simulink model "ClarkAndParkTransforms_harness"  (R2020a)
settings: Solver=VariableStepAuto  StartTime=0.0  StopTime=0.05  RelTol=1e-3
model workspace (MAT data in the model file):
  Vmax = 1
  tol = 1e-09
libraries: ElectricalModelLib x4, simulink x4
settings Model: OrderedModelArguments=off  Creator=cleme  LastModifiedBy=cleme

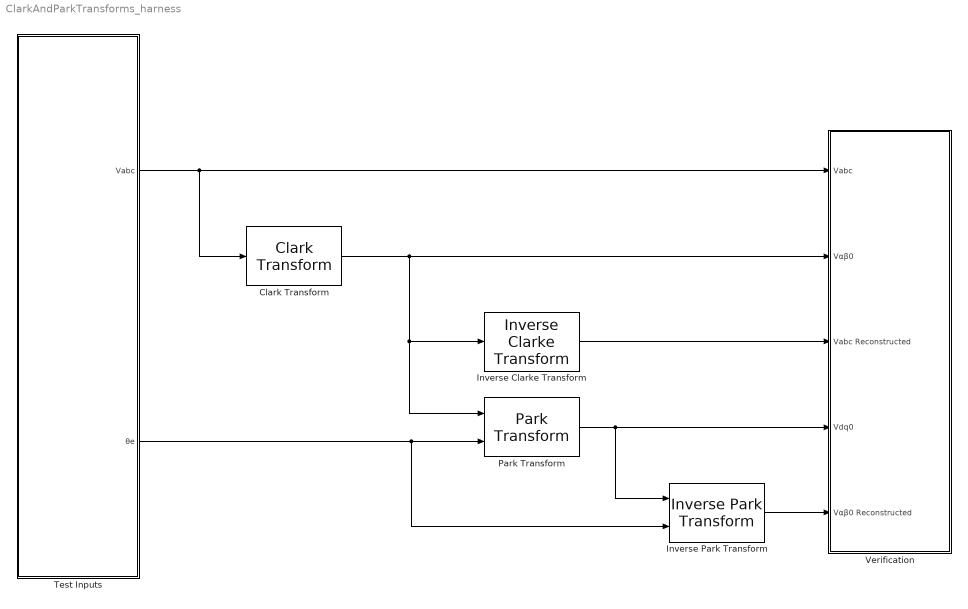
== system ClarkAndParkTransforms_harness ==
  Clark Transform : ElectricalModelLib/Clark Transform
  Inverse Clarke Transform : ElectricalModelLib/Inverse Clarke Transform
  Inverse Park Transform : ElectricalModelLib/Inverse Park Transform
  Park Transform : ElectricalModelLib/Park Transform
  Test Inputs : Subsystem
  Verification : Subsystem
  wires:
  Clark Transform/1 -> Park Transform/1, Inverse Clarke Transform/1, Verification/2(Vαβ0)
  Inverse Clarke Transform/1 -> Verification/3(Vabc Reconstructed)
  Test Inputs/1(Vabc) -> Clark Transform/1, Verification/1(Vabc)
  Test Inputs/2(θe) -> Inverse Park Transform/2, Park Transform/2
  Park Transform/1 -> Verification/4(Vdq0), Inverse Park Transform/1
  Inverse Park Transform/1 -> Verification/5(Vαβ0 Reconstructed)

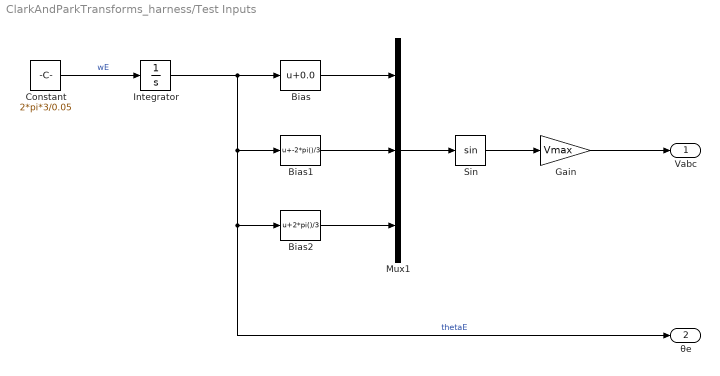
== system ClarkAndParkTransforms_harness/Test Inputs ==
  Bias : Bias  Bias=0.0
  Bias1 : Bias  Bias=-2*pi()/3
  Bias2 : Bias  Bias=2*pi()/3
  Constant : Constant  Value=2*pi*3/0.05
  Gain : Gain  Gain=Vmax
  Integrator : Integrator
  Mux1 : Mux  Inputs=3
  Sin : Trigonometry
  Vabc : Outport
  θe : Outport  Port=2
  wires:
  Sin/1 -> Gain/1
  Constant/1 -> Integrator/1  "wE"
  Integrator/1 -> θe/1, Bias2/1, Bias1/1, Bias/1  "thetaE"
  Bias2/1 -> Mux1/3
  Bias/1 -> Mux1/1
  Bias1/1 -> Mux1/2
  Mux1/1 -> Sin/1
  Gain/1 -> Vabc/1

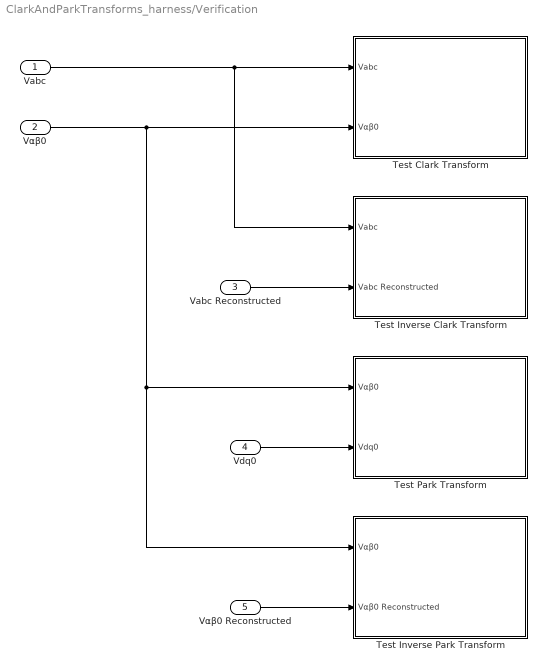
== system ClarkAndParkTransforms_harness/Verification ==
  Vabc : Inport
  Vαβ0 : Inport  Port=2
  Vabc Reconstructed : Inport  Port=3
  Vdq0 : Inport  Port=4
  Vαβ0 Reconstructed : Inport  Port=5
  Test Clark Transform : Subsystem
  Test Inverse Clark Transform : Subsystem
  Test Inverse Park Transform : Subsystem
  Test Park Transform : Subsystem
  wires:
  Vαβ0/1 -> Test Inverse Park Transform/1(Vαβ0), Test Park Transform/1(Vαβ0), Test Clark Transform/2(Vαβ0)
  Vabc/1 -> Test Clark Transform/1(Vabc), Test Inverse Clark Transform/1(Vabc)
  Vabc Reconstructed/1 -> Test Inverse Clark Transform/2(Vabc Reconstructed)
  Vαβ0 Reconstructed/1 -> Test Inverse Park Transform/2(Vαβ0 Reconstructed)
  Vdq0/1 -> Test Park Transform/2(Vdq0)

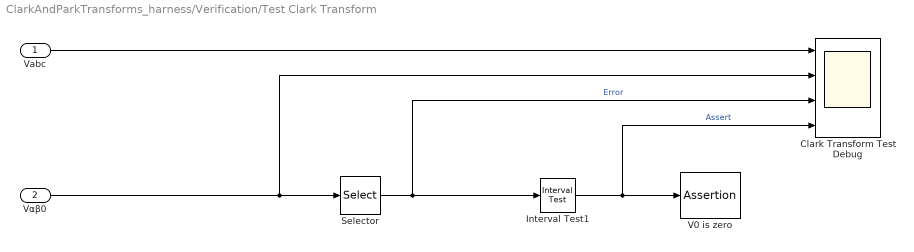
== system ClarkAndParkTransforms_harness/Verification/Test Clark Transform ==
  Vabc : Inport
  Vαβ0 : Inport  Port=2
  Clark Transform Test Debug : Scope  NumInputPorts=4
  Interval Test1 : simulink/Logic and Bit Operations/Interval Test  IntervalClosedRight=on  uplimit=tol  IntervalClosedLeft=on  lowlimit=-tol  OutDataTypeStr=boolean
      settings: AttributesFormatString=|
      | LB = %<lowlimit>
      | UB = %<uplimit>
  Selector : Selector  InputPortWidth=3  IndexOptions=Index vector (dialog)  Indices=3  OutputSizes=1
  V0 is zero : Assertion
  wires:
  Vabc/1 -> Clark Transform Test Debug/1
  Interval Test1/1 -> Clark Transform Test Debug/4, V0 is zero/1  "Assert"
  Vαβ0/1 -> Clark Transform Test Debug/2, Selector/1
  Selector/1 -> Interval Test1/1, Clark Transform Test Debug/3  "Error"

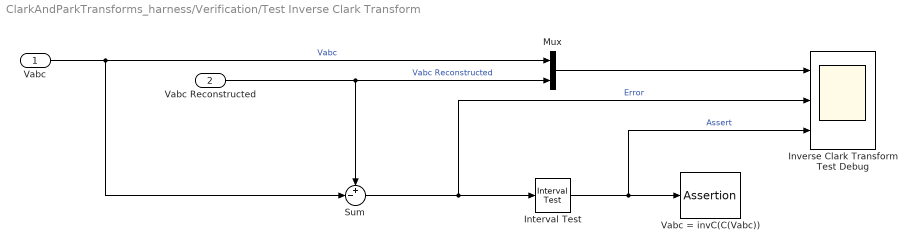
== system ClarkAndParkTransforms_harness/Verification/Test Inverse Clark Transform ==
  Vabc : Inport
  Vabc Reconstructed : Inport  Port=2
  Interval Test : simulink/Logic and Bit Operations/Interval Test  IntervalClosedRight=on  uplimit=tol  IntervalClosedLeft=on  lowlimit=-tol  OutDataTypeStr=boolean
      settings: AttributesFormatString=|
      | LB = %<lowlimit>
      | UB = %<uplimit>
  Inverse Clark Transform Test Debug : Scope  NumInputPorts=3
  Mux : Mux  Inputs=2
  Sum : Sum  Inputs=+-|
  "Vabc = invC(C(Vabc))  " : Assertion
  wires:
  Interval Test/1 -> Inverse Clark Transform Test Debug/3, "Vabc = invC(C(Vabc))  "/1  "Assert"
  Sum/1 -> Interval Test/1, Inverse Clark Transform Test Debug/2  "Error"
  Mux/1 -> Inverse Clark Transform Test Debug/1
  Vabc/1 -> Sum/2, Mux/1  "Vabc"
  Vabc Reconstructed/1 -> Sum/1, Mux/2  "Vabc Reconstructed"

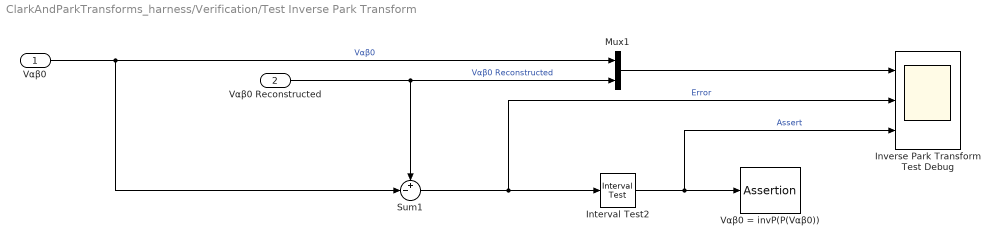
== system ClarkAndParkTransforms_harness/Verification/Test Inverse Park Transform ==
  Vαβ0 : Inport
  Vαβ0 Reconstructed : Inport  Port=2
  Interval Test2 : simulink/Logic and Bit Operations/Interval Test  IntervalClosedRight=on  uplimit=tol  IntervalClosedLeft=on  lowlimit=-tol  OutDataTypeStr=boolean
      settings: AttributesFormatString=|
      | LB = %<lowlimit>
      | UB = %<uplimit>
  Inverse Park Transform Test Debug : Scope  NumInputPorts=3
  Mux1 : Mux  Inputs=2
  Sum1 : Sum  Inputs=+-|
  Vαβ0 = invP(P(Vαβ0)) : Assertion
  wires:
  Interval Test2/1 -> Inverse Park Transform Test Debug/3, Vαβ0 = invP(P(Vαβ0))/1  "Assert"
  Vαβ0 Reconstructed/1 -> Sum1/1, Mux1/2  "Vαβ0 Reconstructed"
  Mux1/1 -> Inverse Park Transform Test Debug/1
  Vαβ0/1 -> Sum1/2, Mux1/1  "Vαβ0"
  Sum1/1 -> Inverse Park Transform Test Debug/2, Interval Test2/1  "Error"

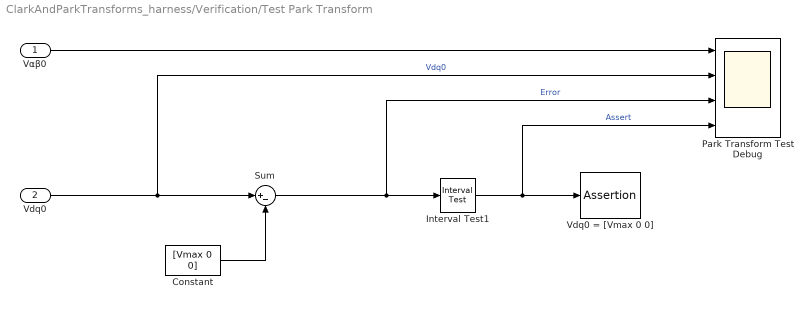
== system ClarkAndParkTransforms_harness/Verification/Test Park Transform ==
  Vαβ0 : Inport
  Vdq0 : Inport  Port=2
  Constant : Constant  Value=[Vmax 0 0]
  Interval Test1 : simulink/Logic and Bit Operations/Interval Test  IntervalClosedRight=on  uplimit=tol  IntervalClosedLeft=on  lowlimit=-tol  OutDataTypeStr=boolean
      settings: AttributesFormatString=|
      | LB = %<lowlimit>
      | UB = %<uplimit>
  Park Transform Test Debug : Scope  NumInputPorts=4
  Sum : Sum  Inputs=|+-
  Vdq0 = [Vmax 0 0] : Assertion
  wires:
  Vdq0/1 -> Sum/1, Park Transform Test Debug/2  "Vdq0"
  Interval Test1/1 -> Park Transform Test Debug/4, Vdq0 = [Vmax 0 0]/1  "Assert"
  Vαβ0/1 -> Park Transform Test Debug/1
  Sum/1 -> Park Transform Test Debug/3, Interval Test1/1  "Error"
  Constant/1 -> Sum/2
